simulink model "fullStateFeadbackWithIntegrator"  (R2024a)
settings: Solver=VariableStepAuto  StartTime=0.0  StopTime=t_sim  RelTol=1e-3
values from neighbouring files (symbols this model uses):
  C = [0 1 1]    [SISO.m]    (also in invertedPendulum.m = [-1 0 0 0; invertedPendulumSys.m = [-1 0 0 0)
  K_q = [-1, -10]    [invertedPendulum.m]    (also in invertedPendulumSys.m)
  K_x = K    [invertedPendulum.m]    (also in invertedPendulumSys.m)
libraries: cstblocks x1
settings Model: Creator=lorenzo  LastModifiedBy=lorenzo

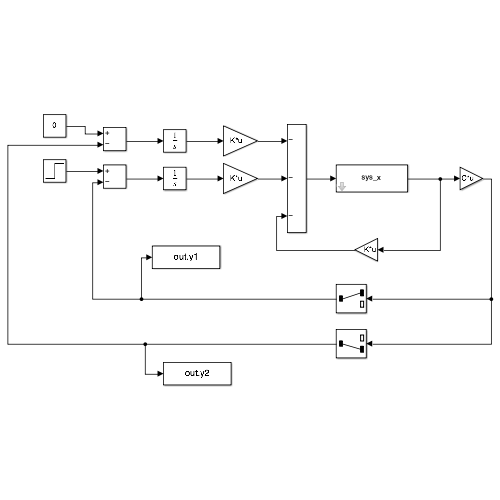
[thumbnail: Simulink's stored preview of the top-level diagram]
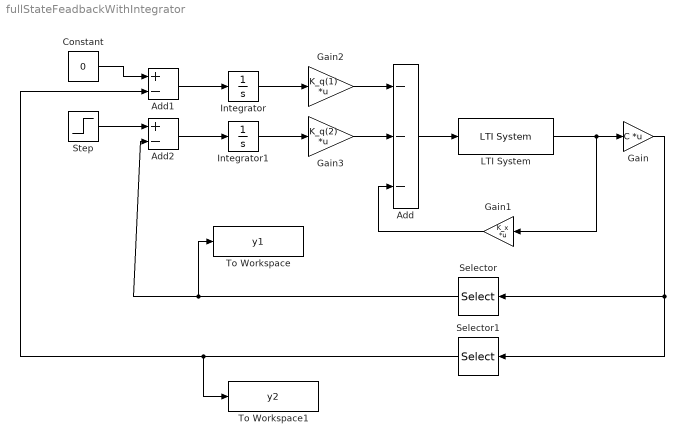
== system fullStateFeadbackWithIntegrator ==
  Add : Sum  Inputs=---
  Add1 : Sum  Inputs=+-
  Add2 : Sum  Inputs=+-
  Constant : Constant  Value=0
  Gain : Gain  Gain=C  Multiplication=Matrix(K*u)
  Gain1 : Gain  Gain=K_x  Multiplication=Matrix(K*u)
  Gain2 : Gain  Gain=K_q(1)  Multiplication=Matrix(K*u)
  Gain3 : Gain  Gain=K_q(2)  Multiplication=Matrix(K*u)
  Integrator : Integrator
  Integrator1 : Integrator
  LTI System : cstblocks/LTI System  sys=sys_x  IC=x0  PadeOrder=0
  Selector : Selector  InputPortWidth=2  IndexOptions=Index vector (dialog)  Indices=1  OutputSizes=1
  Selector1 : Selector  InputPortWidth=2  IndexOptions=Index vector (dialog)  Indices=2  OutputSizes=1
  Step : Step  SampleTime=0
  To Workspace : ToWorkspace  VariableName=y1  SaveFormat=Timeseries  SampleTime=-1
  To Workspace1 : ToWorkspace  VariableName=y2  SaveFormat=Timeseries  SampleTime=-1
  wires:
  Gain/1 -> Selector/1, Selector1/1
  LTI System/1 -> Gain1/1, Gain/1
  Add/1 -> LTI System/1
  Gain2/1 -> Add/1
  Gain1/1 -> Add/3
  Gain3/1 -> Add/2
  Constant/1 -> Add1/1
  Add1/1 -> Integrator/1
  Integrator/1 -> Gain2/1
  Step/1 -> Add2/1
  Add2/1 -> Integrator1/1
  Integrator1/1 -> Gain3/1
  Selector/1 -> To Workspace/1, Add2/2
  Selector1/1 -> To Workspace1/1, Add1/2
